simulink model "rotation_control"  (R2023a)
settings: Solver=FixedStepAuto  StartTime=0.0  StopTime=12  FixedStep=(1/10000)/100  RelTol=1e-3
libraries: simulink x1
settings Model: Creator=lairt  LastModifiedBy=lairt

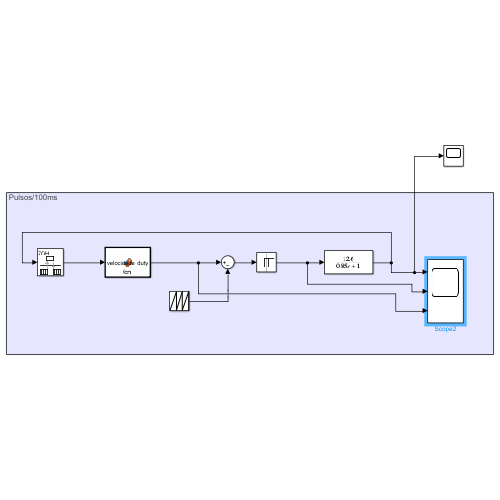
[thumbnail: Simulink's stored preview of the top-level diagram]
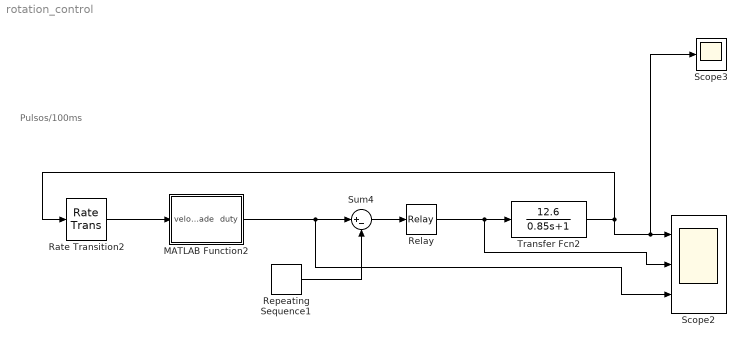
== system rotation_control ==
  note: Pulsos/100ms
  MATLAB Function2 : MATLAB Function  TreatAsAtomicUnit=on
  Rate Transition2 : RateTransition  OutPortSampleTime=0.1
  Relay : Relay  OnOutputValue=5
  Repeating Sequence1 : simulink/Sources/Repeating Sequence  rep_seq_t=[0 1/10000]  rep_seq_y=[0 799]
  Scope2 : Scope  NumInputPorts=3
  Scope3 : Scope
  Sum4 : Sum  Inputs=|+-
  Transfer Fcn2 : TransferFcn  Numerator=[12.6]  Denominator=[0.85 1]
  wires:
  Sum4/1 -> Relay/1
  Repeating Sequence1/1 -> Sum4/2
  Transfer Fcn2/1 -> Rate Transition2/1, Scope3/1, Scope2/1
  Rate Transition2/1 -> MATLAB Function2/1(velocidade)
  MATLAB Function2/1(duty) -> Scope2/3, Sum4/1
  Relay/1 -> Scope2/2, Transfer Fcn2/1

== matlab function rotation_control/MATLAB Function2 ==
  data: velocidade input; duty output
function duty = fcn(velocidade)

persistent ek_1 ek_2 uk_1;

if( isempty(ek_1) ) ek_1=0; end
if( isempty(ek_2) ) ek_2=0; end
if( isempty(uk_1) ) uk_1=0; end

% Erro
vref=40
ek = vref-velocidade


% Controle
% PI
uk = uk_1 + 0.056*(ek - 0.85*ek_1)
% PID
%uk = uk_1 + 0.05*(ek - 1.6*ek_1 + 0.68*ek_2)


% Atraso das variáveis
uk_1=uk
ek_2=ek_1
ek_1=ek

duty = uk*799/5;
